simulink model "pcav"  (R2017b)
settings: Solver=ode2  StartTime=0.0  StopTime=1e-3  FixedStep=1/(fadc*10)  RelTol=1e-3
PreLoadFcn:
  | setup_pcav_simulink
values from neighbouring files (symbols this model uses):
  A = [0, 1 ... (first row only)    [setup_pcav_simulink.m]
  B = [1; 0]    [setup_pcav_simulink.m]
  C = [1 0]    [setup_pcav_simulink.m]
  D = [0]    [setup_pcav_simulink.m]
  fadc = 357e6    (= 357000000)    [cavity_signal.m]    (also in setup_exampleModel_bus_axi_simulink.m; setup_pcav_simulink.m; sysgen_signal.m)
undefined symbols (not defined in the file or in its folder): DiscIntNeverNeededParam
libraries: simulink x7, hdlsllib x1
settings Model: Creator=mitch  LastModifiedBy=charliex
settings DataIOCC: ReturnWorkspaceOutputs=on
settings SFSimCC: SimUseLocalCustomCode=on
settings RTWCC: RTWUseLocalCustomCode=on

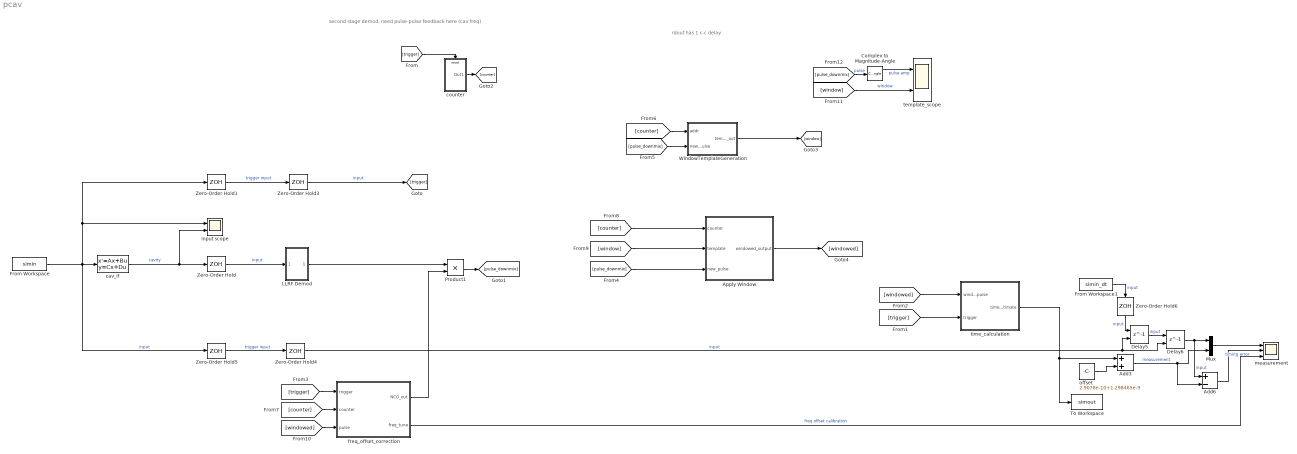
== system pcav ==
  note: rdout has 1 c-c delay
  note: second stage demod, need pulse-pulse feedback here (cav freq)
  Add3 : Sum
  Add6 : Sum  Inputs=+-
  Apply Window : Subsystem
  Complex to Magnitude-Angle : ComplexToMagnitudeAngle
  Delay5 : Delay  DelayLength=1  InitialCondition=0  ShowEnablePort=on
      settings: InputPortMap=u0,e6
  Delay6 : Delay  DelayLength=1  InitialCondition=0  ShowEnablePort=on
      settings: InputPortMap=u0,e6
  From Workspace : FromWorkspace  VariableName=simin  SampleTime=0  OutputAfterFinalValue=Setting to zero
  From Workspace1 : FromWorkspace  VariableName=simin_dt  SampleTime=0  OutputAfterFinalValue=Setting to zero
  LLRF Demod : Subsystem
  Mux : Mux  Inputs=2
  Product1 : Product
  To Workspace : ToWorkspace  VariableName=simout  SaveFormat=Timeseries  SampleTime=-1
  WindowTemplateGeneration : Subsystem
  Zero-Order Hold : ZeroOrderHold  SampleTime=1/fadc
  Zero-Order Hold1 : ZeroOrderHold  SampleTime=1/fadc
  Zero-Order Hold3 : ZeroOrderHold  SampleTime=21/fadc
  Zero-Order Hold4 : ZeroOrderHold  SampleTime=21/fadc
  Zero-Order Hold5 : ZeroOrderHold  SampleTime=1/fadc
  Zero-Order Hold6 : ZeroOrderHold  SampleTime=21/fadc
  cav_if : StateSpace  A=A  B=B  C=C  D=D  InitialCondition=0
  counter : Subsystem
  freq_offset_correction : Subsystem
  input scope : Scope  NumInputPorts=2
  measurement : Scope  NumInputPorts=3
  offset : Constant  Value=2.9078e-10+1.298465e-9  VectorParams1D=off
  template_scope : Scope  NumInputPorts=2
  time_calculation : Subsystem
  wires:
  cav_if/1 -> input scope/2, Zero-Order Hold/1  "cavity"
  From Workspace/1 -> cav_if/1, Zero-Order Hold5/1, input scope/1, Zero-Order Hold1/1  "input"
  Zero-Order Hold/1 -> LLRF Demod/1(In1)  "input"
  Zero-Order Hold3/1 -> [trigger]  "input"
  Zero-Order Hold1/1 -> Zero-Order Hold3/1  "trigger input"
  [trigger] -> counter/Reset
  offset/1 -> Add3/2
  Delay5/1 -> Delay6/1  "input"
  Zero-Order Hold4/1 -> Delay5/2, Delay6/2  "input"
  Zero-Order Hold5/1 -> Zero-Order Hold4/1  "trigger input"
  From Workspace1/1 -> Zero-Order Hold6/1  "input"
  Delay6/1 -> Mux/1, Add6/1  "input"
  Add3/1 -> Add6/2, Mux/2  "measurement"
  Mux/1 -> measurement/1
  Add6/1 -> measurement/2  "timing error"
  Zero-Order Hold6/1 -> Delay5/1  "input"
  Product1/1 -> [pulse_downmix]
  [pulse_downmix] -> WindowTemplateGeneration/2(new_pulse)
  freq_offset_correction/2(freq_tune) -> measurement/3  "freq offset calibration"
  [trigger] -> freq_offset_correction/1(trigger)
  counter/1(Out1) -> [counter]
  [counter] -> WindowTemplateGeneration/1(addr)
  [counter] -> freq_offset_correction/2(counter)
  WindowTemplateGeneration/1(template_out) -> [window]
  time_calculation/1(time_offset_estimate) -> Add3/1, To Workspace/1
  [trigger] -> time_calculation/2(trigger)
  [windowed] -> time_calculation/1(windowed_pulse)
  LLRF Demod/1(demod) -> Product1/1
  freq_offset_correction/1(NCO_out) -> Product1/2
  [windowed] -> freq_offset_correction/3(pulse)
  [window] -> template_scope/2  "window"
  [counter] -> Apply Window/1(counter)
  [window] -> Apply Window/2(template)
  [pulse_downmix] -> Apply Window/3(new_pulse)
  Apply Window/1(windowed_output) -> [windowed]
  [pulse_downmix] -> Complex to Magnitude-Angle/1  "pulse"
  Complex to Magnitude-Angle/1 -> template_scope/1  "pulse amp"

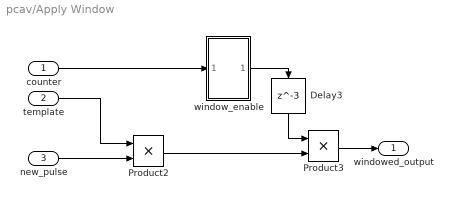
== system pcav/Apply Window ==
  counter : Inport
  template : Inport  Port=2
  new_pulse : Inport  Port=3
  Delay3 : Delay  DelayLength=3  InitialCondition=0
  Product2 : Product
  Product3 : Product
  window_enable : Subsystem
  windowed_output : Outport
  wires:
  new_pulse/1 -> Product2/2
  Delay3/1 -> Product3/1
  Product2/1 -> Product3/2
  Product3/1 -> windowed_output/1
  window_enable/1(Out1) -> Delay3/1
  counter/1 -> window_enable/1(In1)
  template/1 -> Product2/1

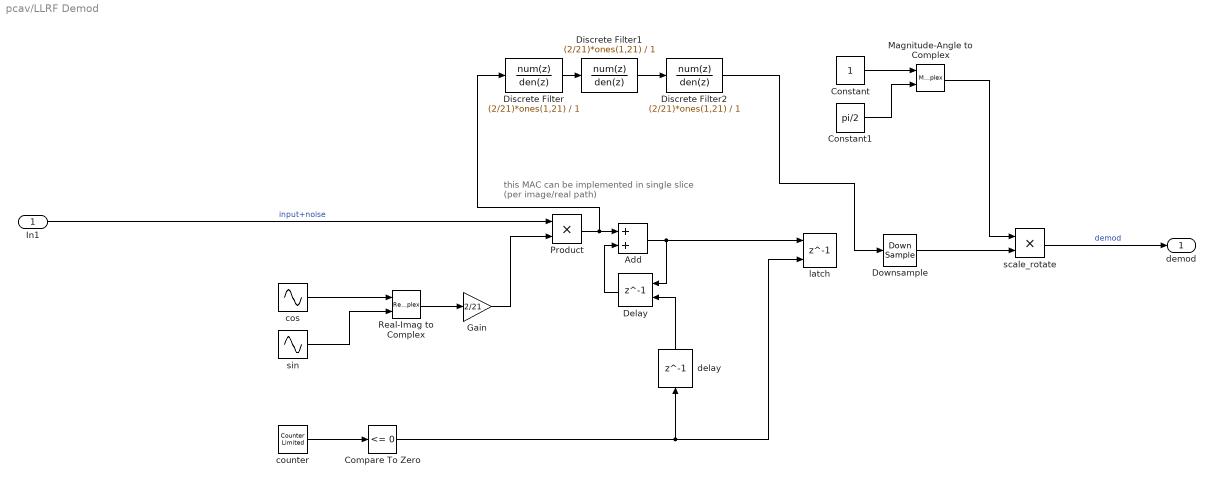
== system pcav/LLRF Demod ==
  note: this MAC can be implemented in single slice
      | (per image/real path)
  In1 : Inport
  Add : Sum
  Compare To Zero : simulink/Logic and Bit Operations/Compare To Zero  relop=<=  OutDataTypeStr=boolean
  Constant : Constant  SampleTime=21/fadc
  Constant1 : Constant  Value=pi/2  SampleTime=21/fadc
  Delay : Delay  DelayLength=1  ExternalReset=Rising
      settings: InputPortMap=u0,r5
  Discrete Filter : DiscreteFilter  Numerator=(2/21)*ones(1,21)  Denominator=1
  Discrete Filter1 : DiscreteFilter  Numerator=(2/21)*ones(1,21)  Denominator=1
  Discrete Filter2 : DiscreteFilter  Numerator=(2/21)*ones(1,21)  Denominator=1
  Downsample : DownSample  N=21  RateOptions=Allow multirate processing
  Gain : Gain  Gain=2/21
  Magnitude-Angle to Complex : MagnitudeAngleToComplex
  Product : Product
  Real-Imag to Complex : RealImagToComplex
  cos : Sin  Frequency=2*pi*85e6  Phase=pi/2  SampleTime=1/fadc
  counter : simulink/Sources/Counter Limited  uplimit=20  tsamp=1/fadc
  delay : Delay  DelayLength=1
  latch : Delay  DelayLength=1  ShowEnablePort=on
      settings: InputPortMap=u0,e6
  scale_rotate : Product
  sin : Sin  Frequency=2*pi*85e6  SampleTime=1/fadc
  demod : Outport
  wires:
  Product/1 -> Discrete Filter/1, Add/1
  cos/1 -> Real-Imag to Complex/1
  Downsample/1 -> scale_rotate/2
  Add/1 -> latch/1, Delay/1
  In1/1 -> Product/1  "input+noise"
  Compare To Zero/1 -> delay/1, latch/2
  scale_rotate/1 -> demod/1  "demod"
  Constant1/1 -> Magnitude-Angle to Complex/2
  Constant/1 -> Magnitude-Angle to Complex/1
  counter/1 -> Compare To Zero/1
  Gain/1 -> Product/2
  Real-Imag to Complex/1 -> Gain/1
  delay/1 -> Delay/2
  sin/1 -> Real-Imag to Complex/2
  Delay/1 -> Add/2
  Magnitude-Angle to Complex/1 -> scale_rotate/1
  Discrete Filter/1 -> Discrete Filter1/1
  Discrete Filter1/1 -> Discrete Filter2/1
  Discrete Filter2/1 -> Downsample/1

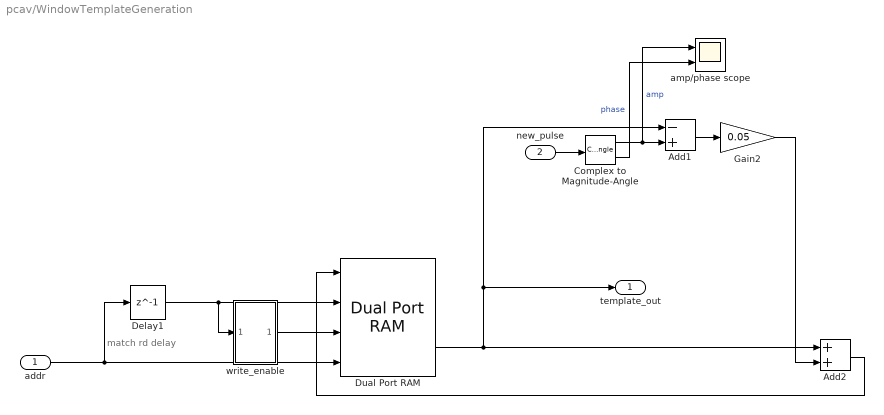
== system pcav/WindowTemplateGeneration ==
  note: match rd delay
  addr : Inport
  new_pulse : Inport  Port=2
  Add1 : Sum  Inputs=-+
  Add2 : Sum
  Complex to Magnitude-Angle : ComplexToMagnitudeAngle
  Delay1 : Delay  DelayLength=1  InitialCondition=0
  Dual Port RAM : hdlsllib/HDL RAMs/Dual Port RAM  ram_size=12
      settings: SourceProductName=Simulink  SourceProductBaseCode=SL
  Gain2 : Gain  Gain=0.05
  amp/phase scope : Scope  NumInputPorts=2
  write_enable : Subsystem
  template_out : Outport
  wires:
  Delay1/1 -> write_enable/1(In1), Dual Port RAM/2
  Gain2/1 -> Add2/2
  Add1/1 -> Gain2/1
  write_enable/1(Out1) -> Dual Port RAM/3
  Add2/1 -> Dual Port RAM/1
  addr/1 -> Dual Port RAM/4, Delay1/1
  Dual Port RAM/2 -> Add1/1, template_out/1, Add2/1
  new_pulse/1 -> Complex to Magnitude-Angle/1
  Complex to Magnitude-Angle/1 -> amp/phase scope/1, Add1/2  "amp"
  Complex to Magnitude-Angle/2 -> amp/phase scope/2  "phase"

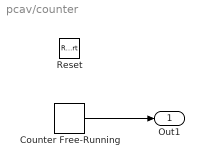
== system pcav/counter ==
  Reset : ResetPort  DisableCoverage=on
  Counter Free-Running : simulink/Sources/Counter Free-Running  NumBits=12  tsamp=21/fadc
  Out1 : Outport
  wires:
  Counter Free-Running/1 -> Out1/1

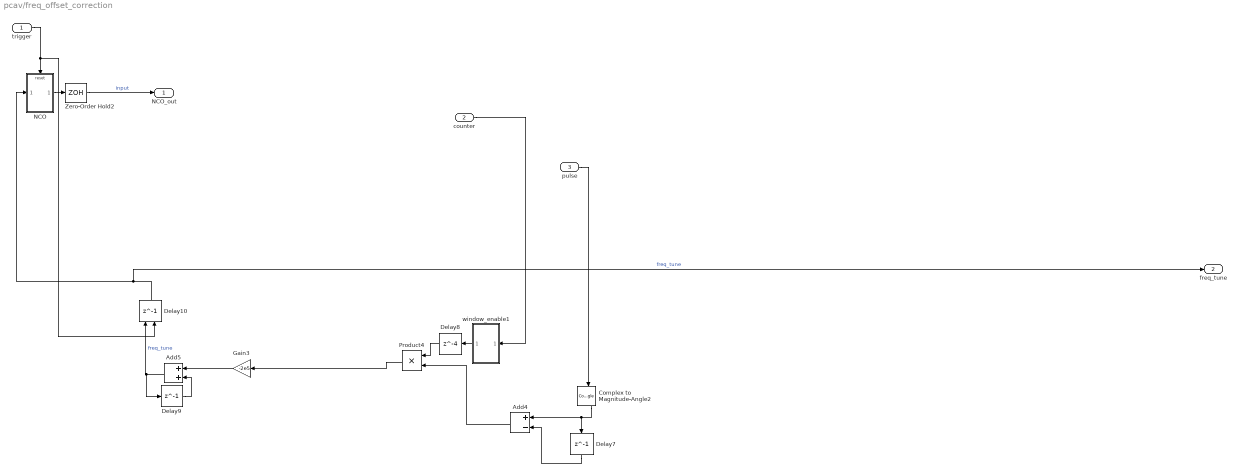
== system pcav/freq_offset_correction ==
  trigger : Inport
  counter : Inport  Port=2
  pulse : Inport  Port=3
  Add4 : Sum  Inputs=+-
  Add5 : Sum
  Complex to Magnitude-Angle2 : ComplexToMagnitudeAngle
  Delay10 : Delay  DelayLength=1  InitialCondition=0  ShowEnablePort=on
      settings: InputPortMap=u0,e6
  Delay7 : Delay  DelayLength=1  InitialCondition=0
  Delay8 : Delay  DelayLength=4  InitialCondition=0
  Delay9 : Delay  DelayLength=1  InitialCondition=0
  Gain3 : Gain  Gain=-2e5
  NCO : Subsystem
  Product4 : Product
  Zero-Order Hold2 : ZeroOrderHold  SampleTime=21/fadc
  window_enable1 : Subsystem
  NCO_out : Outport
  freq_tune : Outport  Port=2
  wires:
  pulse/1 -> Complex to Magnitude-Angle2/1
  counter/1 -> window_enable1/1(In1)
  Delay8/1 -> Product4/1
  Delay10/1 -> freq_tune/1, NCO/1(In1)  "freq_tune"
  Delay9/1 -> Add5/2
  Zero-Order Hold2/1 -> NCO_out/1  "input"
  window_enable1/1(Out1) -> Delay8/1
  Complex to Magnitude-Angle2/2 -> Delay7/1, Add4/1
  Delay7/1 -> Add4/2
  Gain3/1 -> Add5/1
  Add5/1 -> Delay9/1, Delay10/1  "freq_tune"
  Product4/1 -> Gain3/1
  trigger/1 -> Delay10/2, NCO/Reset
  NCO/1(Out1) -> Zero-Order Hold2/1
  Add4/1 -> Product4/2

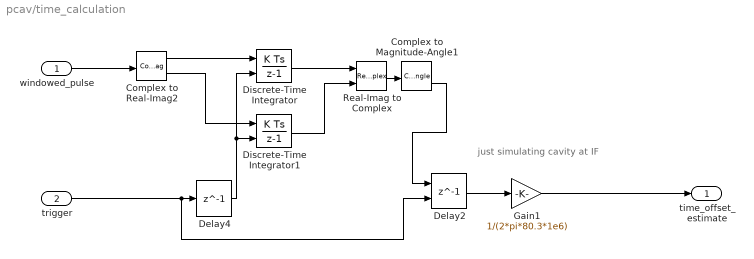
== system pcav/time_calculation ==
  note: just simulating cavity at IF
  windowed_pulse : Inport
  trigger : Inport  Port=2
  Complex to Magnitude-Angle1 : ComplexToMagnitudeAngle
  Complex to Real-Imag2 : ComplexToRealImag
  Delay2 : Delay  DelayLength=1  InitialCondition=0  ShowEnablePort=on
      settings: InputPortMap=u0,e6
  Delay4 : Delay  DelayLength=1  InitialCondition=0
  Discrete-Time Integrator : DiscreteIntegrator  gainval=fadc/21  ExternalReset=rising  InitialConditionSetting=State (most efficient)  SampleTime=-1  ICPrevOutput=DiscIntNeverNeededParam  ICPrevScaledInput=DiscIntNeverNeededParam
  Discrete-Time Integrator1 : DiscreteIntegrator  gainval=fadc/21  ExternalReset=rising  InitialConditionSetting=State (most efficient)  SampleTime=-1  ICPrevOutput=DiscIntNeverNeededParam  ICPrevScaledInput=DiscIntNeverNeededParam
  Gain1 : Gain  Gain=1/(2*pi*80.3*1e6)
  Real-Imag to Complex : RealImagToComplex
  time_offset_estimate : Outport
  wires:
  Complex to Real-Imag2/1 -> Discrete-Time Integrator/1
  Delay4/1 -> Discrete-Time Integrator/2, Discrete-Time Integrator1/2
  Complex to Real-Imag2/2 -> Discrete-Time Integrator1/1
  windowed_pulse/1 -> Complex to Real-Imag2/1
  Discrete-Time Integrator/1 -> Real-Imag to Complex/1
  Gain1/1 -> time_offset_estimate/1
  Delay2/1 -> Gain1/1
  Real-Imag to Complex/1 -> Complex to Magnitude-Angle1/1
  trigger/1 -> Delay2/2, Delay4/1
  Discrete-Time Integrator1/1 -> Real-Imag to Complex/2
  Complex to Magnitude-Angle1/2 -> Delay2/1

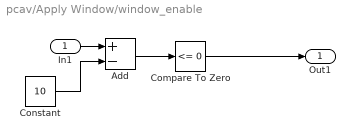
== system pcav/Apply Window/window_enable ==
  In1 : Inport
  Add : Sum  Inputs=+-
  Compare To Zero : simulink/Logic and Bit Operations/Compare To Zero  relop=<=  OutDataTypeStr=boolean
  Constant : Constant  Value=10
  Out1 : Outport
  wires:
  Constant/1 -> Add/2
  Add/1 -> Compare To Zero/1
  In1/1 -> Add/1
  Compare To Zero/1 -> Out1/1

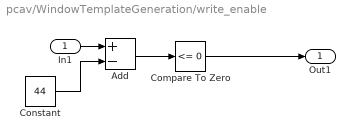
== system pcav/WindowTemplateGeneration/write_enable ==
  In1 : Inport
  Add : Sum  Inputs=+-
  Compare To Zero : simulink/Logic and Bit Operations/Compare To Zero  relop=<=  OutDataTypeStr=boolean
  Constant : Constant  Value=44
  Out1 : Outport
  wires:
  Compare To Zero/1 -> Out1/1
  In1/1 -> Add/1
  Add/1 -> Compare To Zero/1
  Constant/1 -> Add/2

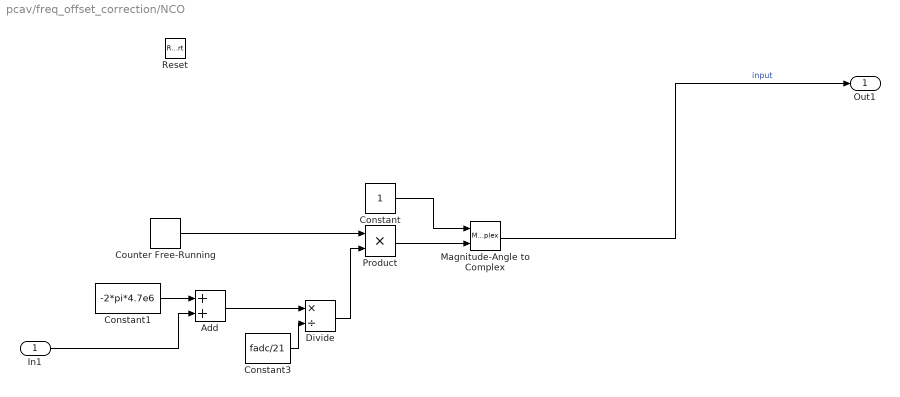
== system pcav/freq_offset_correction/NCO ==
  In1 : Inport
  Reset : ResetPort  DisableCoverage=on
  Add : Sum
  Constant : Constant
  Constant1 : Constant  Value=-2*pi*4.7e6
  Constant3 : Constant  Value=fadc/21
  Counter Free-Running : simulink/Sources/Counter Free-Running  NumBits=32  tsamp=21/fadc
  Divide : Product  Inputs=*/
  Magnitude-Angle to Complex : MagnitudeAngleToComplex
  Product : Product
  Out1 : Outport
  wires:
  Product/1 -> Magnitude-Angle to Complex/2
  Constant3/1 -> Divide/2
  Constant/1 -> Magnitude-Angle to Complex/1
  Divide/1 -> Product/2
  Counter Free-Running/1 -> Product/1
  Constant1/1 -> Add/1
  Add/1 -> Divide/1
  In1/1 -> Add/2
  Magnitude-Angle to Complex/1 -> Out1/1  "input"

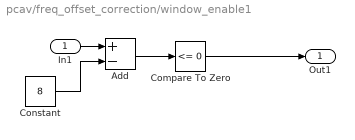
== system pcav/freq_offset_correction/window_enable1 ==
  In1 : Inport
  Add : Sum  Inputs=+-
  Compare To Zero : simulink/Logic and Bit Operations/Compare To Zero  relop=<=  OutDataTypeStr=boolean
  Constant : Constant  Value=8
  Out1 : Outport
  wires:
  Compare To Zero/1 -> Out1/1
  In1/1 -> Add/1
  Add/1 -> Compare To Zero/1
  Constant/1 -> Add/2
